simulink model "water_4hopper_VDF"  (Simulink 8.0)
settings: Solver=ode23t  StartTime=0.0  StopTime=2  MaxStep=1e-2  RelTol=1e-6
undefined symbols (not defined in the file): alpha, amp, b_water, C_d, density, frame_inertia, FRatio, freq, g, K_d, K_i, K_p, K_vir_spring, k_water, leg_length, m_toe, mass, S1, S2, tau, y_0
libraries: mblibv1 x48, powerlib_extras x4, simulink x2
(part 2 of 2)

== system water_4hopper_VDF/leg FR/Subsystem ==
  pos : Inport
  vel : Inport  Port=2
  Constant : Constant  Value=0
  Gain : Gain  Gain=C_d*density
  Gain1 : Gain  Gain=-0.5
  Gain2 : Gain  Gain=S1
  Gain3 : Gain  Gain=g
  Gain4 : Gain  Gain=S2
  Gain5 : Gain  Gain=0.5
  Math Function : Math  Operator=square  SaturateOnIntegerOverflow=on
  Sum : Sum  Inputs=-+|
  Sum1 : Sum  Inputs=-+|
  Switch : Switch  ZeroCross=off
  Switch1 : Switch
  force : Outport
  wires:
  Gain5/1 -> Sum1/2
  Sum1/1 -> Gain2/1
  Constant/1 -> Switch1/1
  Gain/1 -> Switch1/3
  Switch1/1 -> force/1
  Switch/1 -> Gain/1
  Gain2/1 -> Switch/3
  Gain4/1 -> Switch/1
  Sum/1 -> Gain4/1
  Gain3/1 -> Sum1/1, Sum/1
  pos/1 -> Switch1/2, Gain3/1
  Gain1/1 -> Sum/2
  Math Function/1 -> Gain5/1, Gain1/1
  vel/1 -> Math Function/1, Switch/2

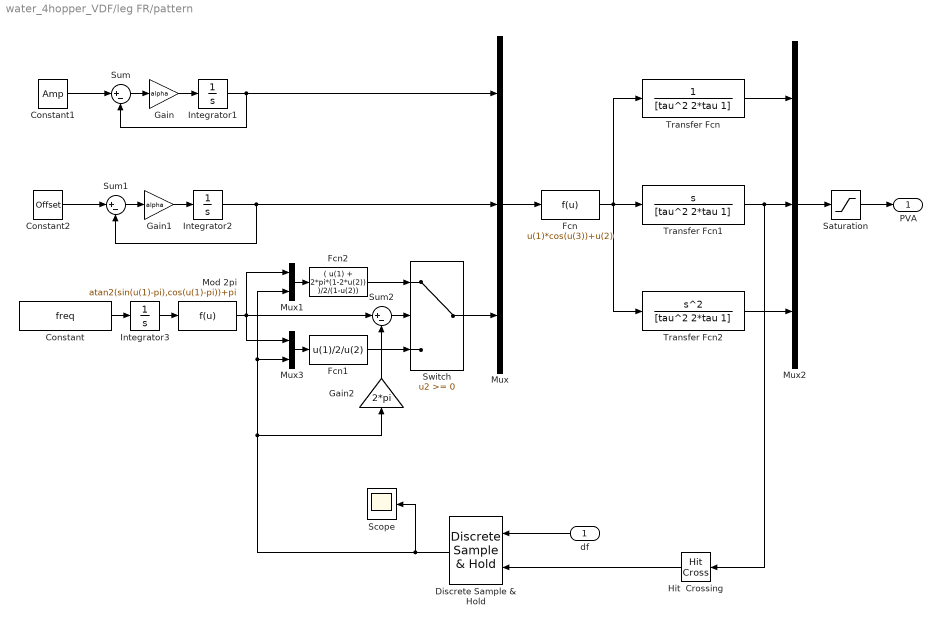
== system water_4hopper_VDF/leg FR/pattern ==
  df : Inport
  Constant : Constant  Value=freq
  Constant1 : Constant  Value=Amp
  Constant2 : Constant  Value=Offset
  Discrete Sample & Hold : powerlib_extras/Discrete  Control Blocks/Discrete Sample & Hold  ic=0.5  Ts=2/pi/freq/20
  Fcn : Fcn  Expr=u(1)*cos(u(3))+u(2)
  Fcn1 : Fcn  Expr=u(1)/2/u(2)
  Fcn2 : Fcn  Expr=( u(1) + 2*pi*(1-2*u(2)) )/2/(1-u(2))
  Gain : Gain  Gain=alpha
  Gain1 : Gain  Gain=alpha
  Gain2 : Gain  Gain=2*pi
  Hit  Crossing : HitCross  HitCrossingDirection=falling
  Integrator1 : Integrator
  Integrator2 : Integrator
  Integrator3 : Integrator  InitialCondition=0.001*rand
  Mod 2pi : Fcn  Expr=atan2(sin(u(1)-pi),cos(u(1)-pi))+pi
  Mux : Mux  Inputs=3
  Mux1 : Mux  Inputs=2
  Mux2 : Mux  Inputs=3
  Mux3 : Mux  Inputs=2
  Saturation : Saturate  UpperLimit=3*amp*freq^2  LowerLimit=-3*amp*freq^2
  Scope : Scope
  Sum : Sum  Inputs=|+-
  Sum1 : Sum  Inputs=|+-
  Sum2 : Sum  Inputs=|+-
  Switch : Switch
  Transfer Fcn : TransferFcn  Denominator=[tau^2 2*tau 1]
  Transfer Fcn1 : TransferFcn  Numerator=[1 0]  Denominator=[tau^2 2*tau 1]
  Transfer Fcn2 : TransferFcn  Numerator=[1 0 0]  Denominator=[tau^2 2*tau 1]
  PVA : Outport
  wires:
  Constant/1 -> Integrator3/1
  Mod 2pi/1 -> Mux1/1, Mux3/1, Sum2/1
  Integrator3/1 -> Mod 2pi/1
  Switch/1 -> Mux/3
  Fcn1/1 -> Switch/3
  Fcn2/1 -> Switch/1
  Mux/1 -> Fcn/1
  Gain1/1 -> Integrator2/1
  Constant2/1 -> Sum1/1
  Integrator2/1 -> Mux/2, Sum1/2
  Sum1/1 -> Gain1/1
  Gain/1 -> Integrator1/1
  Constant1/1 -> Sum/1
  Integrator1/1 -> Mux/1, Sum/2
  Sum/1 -> Gain/1
  Transfer Fcn2/1 -> Mux2/3
  Transfer Fcn/1 -> Mux2/1
  Transfer Fcn1/1 -> Hit  Crossing/1, Mux2/2
  Mux2/1 -> Saturation/1
  Fcn/1 -> Transfer Fcn1/1, Transfer Fcn/1, Transfer Fcn2/1
  Saturation/1 -> PVA/1
  Hit  Crossing/1 -> Discrete Sample & Hold/2
  Sum2/1 -> Switch/2
  Gain2/1 -> Sum2/2
  Discrete Sample & Hold/1 -> Scope/1, Mux3/2, Mux1/2, Gain2/1
  Mux1/1 -> Fcn2/1
  Mux3/1 -> Fcn1/1
  df/1 -> Discrete Sample & Hold/1

== system water_4hopper_VDF/leg HL/Subsystem ==
  pos : Inport
  vel : Inport  Port=2
  Constant : Constant  Value=0
  Gain : Gain  Gain=C_d*density
  Gain1 : Gain  Gain=-0.5
  Gain2 : Gain  Gain=S1
  Gain3 : Gain  Gain=g
  Gain4 : Gain  Gain=S2
  Gain5 : Gain  Gain=0.5
  Math Function : Math  Operator=square  SaturateOnIntegerOverflow=on
  Sum : Sum  Inputs=-+|
  Sum1 : Sum  Inputs=-+|
  Switch : Switch  ZeroCross=off
  Switch1 : Switch
  force : Outport
  wires:
  Gain5/1 -> Sum1/2
  Sum1/1 -> Gain2/1
  Constant/1 -> Switch1/1
  Gain/1 -> Switch1/3
  Switch1/1 -> force/1
  Switch/1 -> Gain/1
  Gain2/1 -> Switch/3
  Gain4/1 -> Switch/1
  Sum/1 -> Gain4/1
  Gain3/1 -> Sum1/1, Sum/1
  pos/1 -> Switch1/2, Gain3/1
  Gain1/1 -> Sum/2
  Math Function/1 -> Gain5/1, Gain1/1
  vel/1 -> Math Function/1, Switch/2

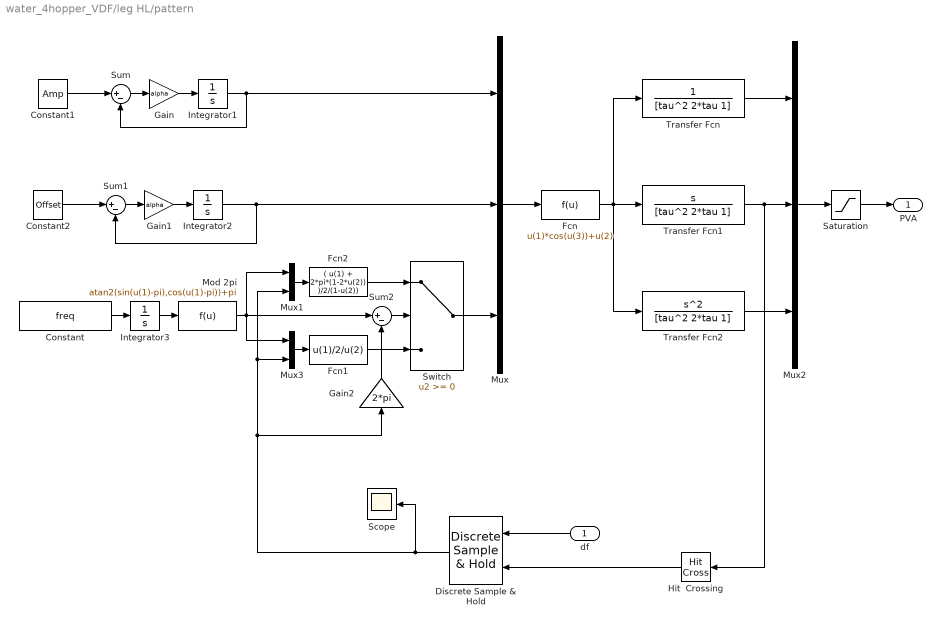
== system water_4hopper_VDF/leg HL/pattern ==
  df : Inport
  Constant : Constant  Value=freq
  Constant1 : Constant  Value=Amp
  Constant2 : Constant  Value=Offset
  Discrete Sample & Hold : powerlib_extras/Discrete  Control Blocks/Discrete Sample & Hold  ic=0.5  Ts=2/pi/freq/20
  Fcn : Fcn  Expr=u(1)*cos(u(3))+u(2)
  Fcn1 : Fcn  Expr=u(1)/2/u(2)
  Fcn2 : Fcn  Expr=( u(1) + 2*pi*(1-2*u(2)) )/2/(1-u(2))
  Gain : Gain  Gain=alpha
  Gain1 : Gain  Gain=alpha
  Gain2 : Gain  Gain=2*pi
  Hit  Crossing : HitCross  HitCrossingDirection=falling
  Integrator1 : Integrator
  Integrator2 : Integrator
  Integrator3 : Integrator  InitialCondition=0.001*rand
  Mod 2pi : Fcn  Expr=atan2(sin(u(1)-pi),cos(u(1)-pi))+pi
  Mux : Mux  Inputs=3
  Mux1 : Mux  Inputs=2
  Mux2 : Mux  Inputs=3
  Mux3 : Mux  Inputs=2
  Saturation : Saturate  UpperLimit=3*amp*freq^2  LowerLimit=-3*amp*freq^2
  Scope : Scope
  Sum : Sum  Inputs=|+-
  Sum1 : Sum  Inputs=|+-
  Sum2 : Sum  Inputs=|+-
  Switch : Switch
  Transfer Fcn : TransferFcn  Denominator=[tau^2 2*tau 1]
  Transfer Fcn1 : TransferFcn  Numerator=[1 0]  Denominator=[tau^2 2*tau 1]
  Transfer Fcn2 : TransferFcn  Numerator=[1 0 0]  Denominator=[tau^2 2*tau 1]
  PVA : Outport
  wires:
  Constant/1 -> Integrator3/1
  Mod 2pi/1 -> Mux1/1, Mux3/1, Sum2/1
  Integrator3/1 -> Mod 2pi/1
  Switch/1 -> Mux/3
  Fcn1/1 -> Switch/3
  Fcn2/1 -> Switch/1
  Mux/1 -> Fcn/1
  Gain1/1 -> Integrator2/1
  Constant2/1 -> Sum1/1
  Integrator2/1 -> Mux/2, Sum1/2
  Sum1/1 -> Gain1/1
  Gain/1 -> Integrator1/1
  Constant1/1 -> Sum/1
  Integrator1/1 -> Mux/1, Sum/2
  Sum/1 -> Gain/1
  Transfer Fcn2/1 -> Mux2/3
  Transfer Fcn/1 -> Mux2/1
  Transfer Fcn1/1 -> Hit  Crossing/1, Mux2/2
  Mux2/1 -> Saturation/1
  Fcn/1 -> Transfer Fcn1/1, Transfer Fcn/1, Transfer Fcn2/1
  Saturation/1 -> PVA/1
  Hit  Crossing/1 -> Discrete Sample & Hold/2
  Sum2/1 -> Switch/2
  Gain2/1 -> Sum2/2
  Discrete Sample & Hold/1 -> Scope/1, Mux3/2, Mux1/2, Gain2/1
  Mux1/1 -> Fcn2/1
  Mux3/1 -> Fcn1/1
  df/1 -> Discrete Sample & Hold/1

== system water_4hopper_VDF/leg HR/Subsystem ==
  pos : Inport
  vel : Inport  Port=2
  Constant : Constant  Value=0
  Gain : Gain  Gain=C_d*density
  Gain1 : Gain  Gain=-0.5
  Gain2 : Gain  Gain=S1
  Gain3 : Gain  Gain=g
  Gain4 : Gain  Gain=S2
  Gain5 : Gain  Gain=0.5
  Math Function : Math  Operator=square  SaturateOnIntegerOverflow=on
  Sum : Sum  Inputs=-+|
  Sum1 : Sum  Inputs=-+|
  Switch : Switch  ZeroCross=off
  Switch1 : Switch
  force : Outport
  wires:
  Gain5/1 -> Sum1/2
  Sum1/1 -> Gain2/1
  Constant/1 -> Switch1/1
  Gain/1 -> Switch1/3
  Switch1/1 -> force/1
  Switch/1 -> Gain/1
  Gain2/1 -> Switch/3
  Gain4/1 -> Switch/1
  Sum/1 -> Gain4/1
  Gain3/1 -> Sum1/1, Sum/1
  pos/1 -> Switch1/2, Gain3/1
  Gain1/1 -> Sum/2
  Math Function/1 -> Gain5/1, Gain1/1
  vel/1 -> Math Function/1, Switch/2

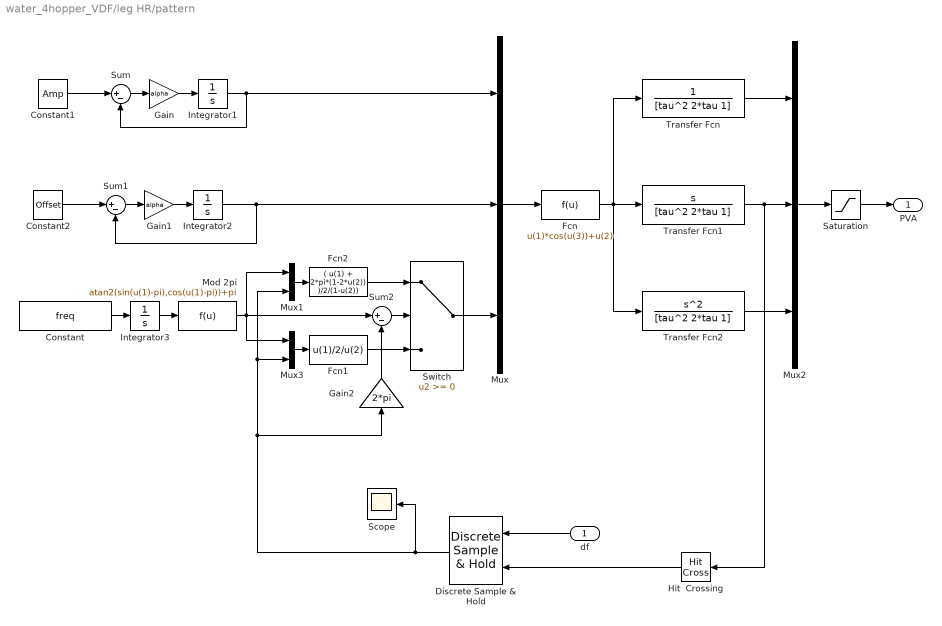
== system water_4hopper_VDF/leg HR/pattern ==
  df : Inport
  Constant : Constant  Value=freq
  Constant1 : Constant  Value=Amp
  Constant2 : Constant  Value=Offset
  Discrete Sample & Hold : powerlib_extras/Discrete  Control Blocks/Discrete Sample & Hold  ic=0.5  Ts=2/pi/freq/20
  Fcn : Fcn  Expr=u(1)*cos(u(3))+u(2)
  Fcn1 : Fcn  Expr=u(1)/2/u(2)
  Fcn2 : Fcn  Expr=( u(1) + 2*pi*(1-2*u(2)) )/2/(1-u(2))
  Gain : Gain  Gain=alpha
  Gain1 : Gain  Gain=alpha
  Gain2 : Gain  Gain=2*pi
  Hit  Crossing : HitCross  HitCrossingDirection=falling
  Integrator1 : Integrator
  Integrator2 : Integrator
  Integrator3 : Integrator  InitialCondition=pi
  Mod 2pi : Fcn  Expr=atan2(sin(u(1)-pi),cos(u(1)-pi))+pi
  Mux : Mux  Inputs=3
  Mux1 : Mux  Inputs=2
  Mux2 : Mux  Inputs=3
  Mux3 : Mux  Inputs=2
  Saturation : Saturate  UpperLimit=3*amp*freq^2  LowerLimit=-3*amp*freq^2
  Scope : Scope
  Sum : Sum  Inputs=|+-
  Sum1 : Sum  Inputs=|+-
  Sum2 : Sum  Inputs=|+-
  Switch : Switch
  Transfer Fcn : TransferFcn  Denominator=[tau^2 2*tau 1]
  Transfer Fcn1 : TransferFcn  Numerator=[1 0]  Denominator=[tau^2 2*tau 1]
  Transfer Fcn2 : TransferFcn  Numerator=[1 0 0]  Denominator=[tau^2 2*tau 1]
  PVA : Outport
  wires:
  Constant/1 -> Integrator3/1
  Mod 2pi/1 -> Mux1/1, Mux3/1, Sum2/1
  Integrator3/1 -> Mod 2pi/1
  Switch/1 -> Mux/3
  Fcn1/1 -> Switch/3
  Fcn2/1 -> Switch/1
  Mux/1 -> Fcn/1
  Gain1/1 -> Integrator2/1
  Constant2/1 -> Sum1/1
  Integrator2/1 -> Mux/2, Sum1/2
  Sum1/1 -> Gain1/1
  Gain/1 -> Integrator1/1
  Constant1/1 -> Sum/1
  Integrator1/1 -> Mux/1, Sum/2
  Sum/1 -> Gain/1
  Transfer Fcn2/1 -> Mux2/3
  Transfer Fcn/1 -> Mux2/1
  Transfer Fcn1/1 -> Hit  Crossing/1, Mux2/2
  Mux2/1 -> Saturation/1
  Fcn/1 -> Transfer Fcn1/1, Transfer Fcn/1, Transfer Fcn2/1
  Saturation/1 -> PVA/1
  Hit  Crossing/1 -> Discrete Sample & Hold/2
  Sum2/1 -> Switch/2
  Gain2/1 -> Sum2/2
  Discrete Sample & Hold/1 -> Scope/1, Mux3/2, Mux1/2, Gain2/1
  Mux1/1 -> Fcn2/1
  Mux3/1 -> Fcn1/1
  df/1 -> Discrete Sample & Hold/1

== matlab function PID 1/MATLAB Function ==
  data: u input double; y output double
 function y = fcn(u)

mass = 0.1/4;
leg_length = 0.0249;
A = leg_length;
omega = 60;
forceRatio = 1/16;

h = u(1)-leg_length;
DF = u(2);



r1 = 0.02;
S1 = pi*r1^2*0.9185;
density = 1000;
g = 9.81;
C_d = 0.703;

b = 0.5*C_d*S1*density;
k = C_d*S1*density*g;
W = mass*g;

if h > A, h = A;end
if h < -A, h = -A;end

 
%F = (omega^2*b/(8*pi)*((pi/2 - asin(h/A))*A^2 - h*sqrt(A^2 - h^2))*(1/DF - forceRatio/(1-DF)) ...
%    - k/(pi)*((pi/2 - asin(h/A))*h - sqrt(A^2 - h^2))*(DF + forceRatio*(1-DF))) - W;

DF_0 = DF;
F_ap = (omega^2*b/(8*pi)*((pi/2 - asin(h/A))*A^2 - h*sqrt(A^2 - h^2))*((1/DF_0-forceRatio/(1-DF_0)) + ( -DF_0^-2 - forceRatio*(1-DF_0)^-2)*(DF - DF_0)) ...
    - k/(pi)*((pi/2 - asin(h/A))*h - sqrt(A^2 - h^2))*(DF + forceRatio*(1-DF))) - W;



y = F_ap;

== matlab function PID 2/MATLAB Function ==
  data: u input double; y output double
 function y = fcn(u)

mass = 0.1/4;
leg_length = 0.0249;
A = leg_length;
omega = 60;
forceRatio = 1/16;

h = u(1)-leg_length;
DF = u(2);



r1 = 0.02;
S1 = pi*r1^2*0.9185;
density = 1000;
g = 9.81;
C_d = 0.703;

b = 0.5*C_d*S1*density;
k = C_d*S1*density*g;
W = mass*g;

if h > A, h = A;end
if h < -A, h = -A;end

 
%F = (omega^2*b/(8*pi)*((pi/2 - asin(h/A))*A^2 - h*sqrt(A^2 - h^2))*(1/DF - forceRatio/(1-DF)) ...
%    - k/(pi)*((pi/2 - asin(h/A))*h - sqrt(A^2 - h^2))*(DF + forceRatio*(1-DF))) - W;

DF_0 = DF;
F_ap = (omega^2*b/(8*pi)*((pi/2 - asin(h/A))*A^2 - h*sqrt(A^2 - h^2))*((1/DF_0-forceRatio/(1-DF_0)) + ( -DF_0^-2 - forceRatio*(1-DF_0)^-2)*(DF - DF_0)) ...
    - k/(pi)*((pi/2 - asin(h/A))*h - sqrt(A^2 - h^2))*(DF + forceRatio*(1-DF))) - W;



y = F_ap;
